simulink model "main_chua_sim_2014a"  (R2014a)
settings: Solver=ode45  SolverMode=SingleTasking  StartTime=0.0  StopTime=tfin  FixedStep=0.1  RelTol=1e-3
values from neighbouring files (symbols this model uses):
  a = 10.4    [main_chua.m]
  b = 16.5    [main_chua.m]
  C = [1 0 0]    [main_chua.m]
  R = 0.1    [main_chua.m]
  x0 = randn(3,1)*0    [main_chua.m]
undefined symbols (not defined in the file or in its folder): mu_chua, r, ref_chua, rho_chua, u_chua
settings Model: CovMetricSettings=dwe  CovHtmlReporting=off  covSaveCumulativeToWorkspaceVar=off  CovSaveSingleToWorkspaceVar=off  CovExternalEMLEnable=on  CovSFcnEnable=on  Creator=carlonovara  LastModifiedBy=carlonovara
settings DataIOCC: LimitDataPoints=off  SaveFormat=StructureWithTime
settings DebuggingCC: MergeDetectMultiDrivingBlocksExec=error  SolverPrmCheckMsg=none  FrameProcessingCompatibilityMsg=error  SFUnexpectedBacktrackingDiag=error  SFNoUnconditionalDefaultTransitionDiag=error
settings HardwareCC: ProdBitPerPointer=64  ProdLargestAtomicFloat=Float  ProdIntDivRoundTo=Zero  ProdEndianess=LittleEndian  ProdHWDeviceType=Specified
settings ModelReferenceCC: PropagateSignalLabelsOutOfModel=on
settings GRTTargetCC: TargetLangStandard=C99 (ISO)  GeneratePreprocessorConditionals=Use local settings

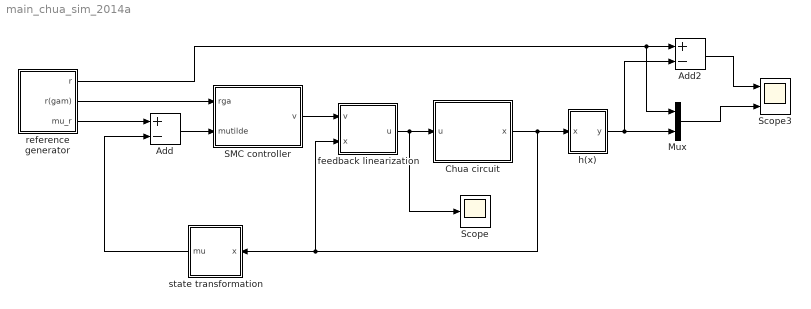
== system main_chua_sim_2014a ==
  Add : Sum  Inputs=+-
  Add2 : Sum  Inputs=+-
  Chua circuit : Subsystem
  Mux : Mux  Inputs=2
  SMC controller : MATLAB Function  TreatAsAtomicUnit=on
      settings: PermitHierarchicalResolution=ParametersOnly
  Scope : Scope
      settings: TimeRange=auto  MaxDataPoints=5000  SaveToWorkspace=off  YMin=-6.86087  YMax=7.13829  SampleTime=-1
  Scope3 : Scope  NumInputPorts=2
      settings: TimeRange=auto  MaxDataPoints=5000  SaveToWorkspace=off  YMin=-3.36955~-3.375  YMax=0.32594~0.375  SampleTime=-1
  feedback linearization : Subsystem
  h(x) : Subsystem
  reference generator : Subsystem
  state transformation : Subsystem
  wires:
  Chua circuit/1(x) -> h(x)/1(x), feedback linearization/2(x), state transformation/1(x)
  h(x)/1(y) -> Mux/2, Add2/2
  reference generator/3(mu_r) -> Add/1
  state transformation/1(mu) -> Add/2
  reference generator/1(r) -> Mux/1, Add2/1
  reference generator/2(r(gam)) -> SMC controller/1(rga)
  Add/1 -> SMC controller/2(mutilde)
  Add2/1 -> Scope3/1
  Mux/1 -> Scope3/2
  feedback linearization/1(u) -> Scope/1, Chua circuit/1(u)
  SMC controller/1(v) -> feedback linearization/1(v)

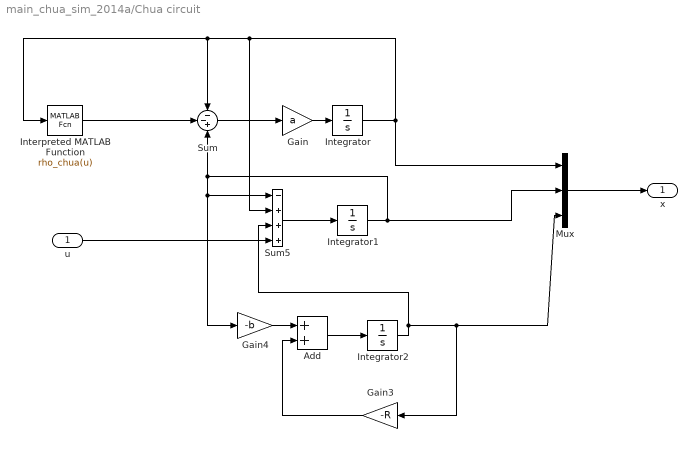
== system main_chua_sim_2014a/Chua circuit ==
  u : Inport
  Add : Sum
  Gain : Gain  Gain=a
  Gain3 : Gain  Gain=-R
  Gain4 : Gain  Gain=-b
  Integrator : Integrator  InitialCondition=x0(1)
  Integrator1 : Integrator  InitialCondition=x0(2)
  Integrator2 : Integrator  InitialCondition=x0(3)
  Interpreted MATLAB Function : MATLABFcn  MATLABFcn=rho_chua(u)
  Mux : Mux  Inputs=3
  Sum : Sum  Inputs=--+
  Sum5 : Sum  Inputs=-+++
  x : Outport
  wires:
  Sum/1 -> Gain/1
  Gain/1 -> Integrator/1
  Integrator1/1 -> Mux/2, Sum5/1, Gain4/1, Sum/3
  Sum5/1 -> Integrator1/1
  Integrator2/1 -> Gain3/1, Mux/3, Sum5/3
  Mux/1 -> x/1
  Gain4/1 -> Add/1
  Add/1 -> Integrator2/1
  Gain3/1 -> Add/2
  Integrator/1 -> Mux/1, Sum5/2, Sum/1, Interpreted MATLAB Function/1
  Interpreted MATLAB Function/1 -> Sum/2
  u/1 -> Sum5/4

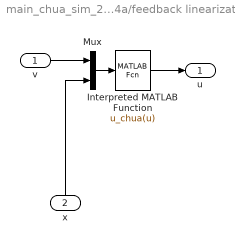
== system main_chua_sim_2014a/feedback linearization ==
  v : Inport
  x : Inport  Port=2
  Interpreted MATLAB Function : MATLABFcn  MATLABFcn=u_chua(u)
  Mux : Mux  Inputs=2
  u : Outport
  wires:
  x/1 -> Mux/2
  Mux/1 -> Interpreted MATLAB Function/1
  Interpreted MATLAB Function/1 -> u/1
  v/1 -> Mux/1

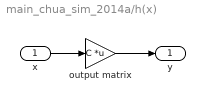
== system main_chua_sim_2014a/h(x) ==
  x : Inport
  output matrix : Gain  Gain=C  Multiplication=Matrix(K*u)
  y : Outport
  wires:
  x/1 -> output matrix/1
  output matrix/1 -> y/1

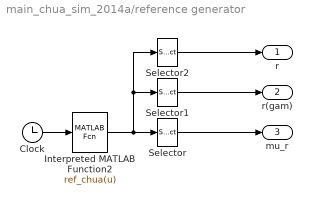
== system main_chua_sim_2014a/reference generator ==
  Clock : Clock
  Interpreted MATLAB Function2 : MATLABFcn  MATLABFcn=ref_chua(u)
  Selector : Selector  InputPortWidth=r+1  IndexOptions=Index vector (dialog)  Indices=1:r  OutputSizes=1
  Selector1 : Selector  InputPortWidth=r+1  IndexOptions=Index vector (dialog)  Indices=r+1  OutputSizes=1
  Selector2 : Selector  InputPortWidth=r+1  IndexOptions=Index vector (dialog)  Indices=1  OutputSizes=1
  r : Outport
  r(gam) : Outport  Port=2
  mu_r : Outport  Port=3
  wires:
  Clock/1 -> Interpreted MATLAB Function2/1
  Selector1/1 -> r(gam)/1
  Selector2/1 -> r/1
  Interpreted MATLAB Function2/1 -> Selector2/1, Selector1/1, Selector/1
  Selector/1 -> mu_r/1

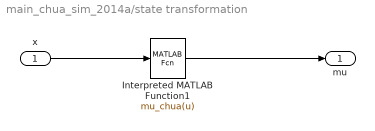
== system main_chua_sim_2014a/state transformation ==
  x : Inport
  Interpreted MATLAB Function1 : MATLABFcn  MATLABFcn=mu_chua(u)
  mu : Outport
  wires:
  x/1 -> Interpreted MATLAB Function1/1
  Interpreted MATLAB Function1/1 -> mu/1

== matlab function main_chua_sim_2014a/SMC controller ==
  data: rga input; v output; mutilde input
function v=smc_chua(rga,mutilde)

% parameters
k1=80;
k2=50;

if 1

eta=1;

% sliding surface function
s=mutilde(2)+k2*mutilde(1);

% sliding mode control law
% v=rga+k2*mutilde(2)+k1*sign(s);
v=rga+k2*mutilde(2)+k1*tanh(eta*s);

else

% feedback linearization control law
v=rga+k2*mutilde(2)+k1*mutilde(1);

end
